simulink model "fault_detection_system"  (R2025b)
settings: Solver=ode4  StartTime=0.0  StopTime=120  FixedStep=0.01  RelTol=1e-3
settings Model: Creator=Santy  LastModifiedBy=Santy
settings DataIOCC: SignalLogging=off  DSMLogging=off  ReturnWorkspaceOutputs=off

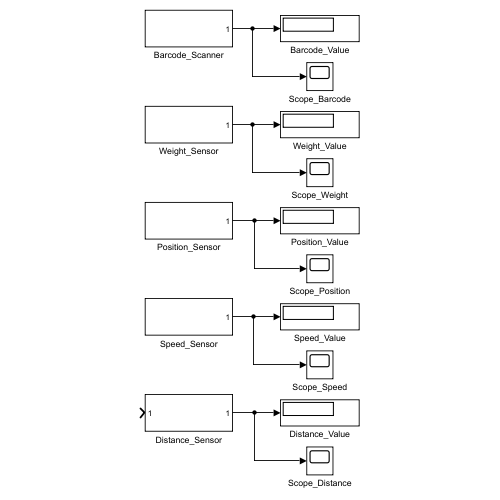
[thumbnail: Simulink's stored preview of the top-level diagram]
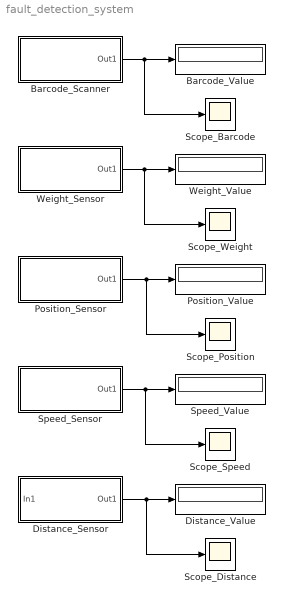
== system fault_detection_system ==
  Barcode_Scanner : Subsystem
  Barcode_Value : Display
  Distance_Sensor : Subsystem
  Distance_Value : Display
  Position_Sensor : Subsystem
  Position_Value : Display
  Scope_Barcode : Scope
  Scope_Distance : Scope
      settings: ActiveDisplayYMinimum=5.925579144887446  ActiveDisplayYMaximum=24.55859374233901  DataLoggingVariableName=ScopeData5
  Scope_Position : Scope
      settings: ActiveDisplayYMinimum=-1  ActiveDisplayYMaximum=1  DataLoggingVariableName=ScopeData3
  Scope_Speed : Scope
      settings: ActiveDisplayYMinimum=1.28548947418835  ActiveDisplayYMaximum=1.7495442770751002  DataLoggingVariableName=ScopeData4
  Scope_Weight : Scope
      settings: DataLoggingVariableName=ScopeData2
  Speed_Sensor : Subsystem
  Speed_Value : Display
  Weight_Sensor : Subsystem
  Weight_Value : Display
  wires:
  Barcode_Scanner/1(Out1) -> Scope_Barcode/1, Barcode_Value/1
  Weight_Sensor/1(Out1) -> Scope_Weight/1, Weight_Value/1
  Position_Sensor/1(Out1) -> Scope_Position/1, Position_Value/1
  Speed_Sensor/1(Out1) -> Scope_Speed/1, Speed_Value/1
  Distance_Sensor/1(Out1) -> Scope_Distance/1, Distance_Value/1

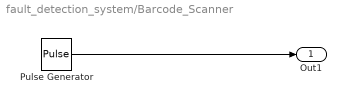
== system fault_detection_system/Barcode_Scanner ==
  Pulse Generator : DiscretePulseGenerator  Period=800  PulseWidth=10  SampleTime=0.01
  Out1 : Outport
  wires:
  Pulse Generator/1 -> Out1/1

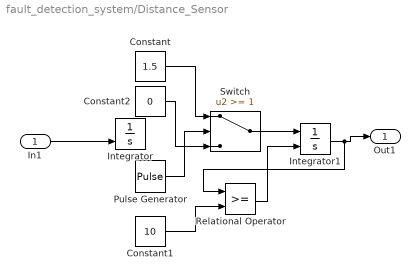
== system fault_detection_system/Distance_Sensor ==
  In1 : Inport
  Constant : Constant  Value=1.5
  Constant1 : Constant  Value=10
  Constant2 : Constant  Value=0
  Integrator : Integrator  ExternalReset=rising
  Integrator1 : Integrator  ExternalReset=rising
  Pulse Generator : DiscretePulseGenerator  Amplitude=10  Period=800  PulseWidth=667  SampleTime=0.01
  Relational Operator : RelationalOperator  OutDataTypeStr=boolean  RndMeth=Simplest  InputSameDT=off
  Switch : Switch  Threshold=1  SaturateOnIntegerOverflow=off  InputSameDT=off
  Out1 : Outport
  wires:
  In1/1 -> Integrator/2
  Pulse Generator/1 -> Switch/2
  Constant/1 -> Switch/1
  Integrator1/1 -> Relational Operator/1, Out1/1
  Constant1/1 -> Relational Operator/2
  Relational Operator/1 -> Integrator1/2
  Switch/1 -> Integrator1/1
  Constant2/1 -> Switch/3

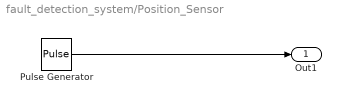
== system fault_detection_system/Position_Sensor ==
  Pulse Generator : DiscretePulseGenerator  Period=800  PulseWidth=667  SampleTime=0.01
  Out1 : Outport
  wires:
  Pulse Generator/1 -> Out1/1

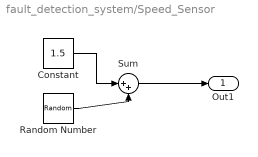
== system fault_detection_system/Speed_Sensor ==
  Constant : Constant  Value=1.5
  Random Number : RandomNumber  Variance=0.0025  Seed=9999  SampleTime=0.01
  Sum : Sum  Inputs=|++
  Out1 : Outport
  wires:
  Sum/1 -> Out1/1
  Random Number/1 -> Sum/2
  Constant/1 -> Sum/1

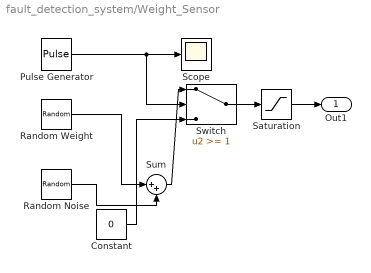
== system fault_detection_system/Weight_Sensor ==
  Constant : Constant  Value=0
  Pulse Generator : DiscretePulseGenerator  Period=800  PulseWidth=80  SampleTime=0.01
  Random Noise : RandomNumber  Variance=0.25  Seed=5678  SampleTime=0.01
  Random Weight : RandomNumber  Mean=25  Variance=64  Seed=1234  SampleTime=0.1
  Saturation : Saturate  UpperLimit=50  LowerLimit=0
  Scope : Scope
      settings: ActiveDisplayYMinimum=-1  ActiveDisplayYMaximum=1
  Sum : Sum  Inputs=|++
  Switch : Switch  Threshold=1  SaturateOnIntegerOverflow=off  InputSameDT=off
  Out1 : Outport
  wires:
  Pulse Generator/1 -> Scope/1, Switch/2
  Random Weight/1 -> Sum/1
  Random Noise/1 -> Sum/2
  Sum/1 -> Switch/1
  Constant/1 -> Switch/3
  Switch/1 -> Saturation/1
  Saturation/1 -> Out1/1
